simulink model "SIMULINK_1-03"  (R2024b)
settings: Solver=ode45  StartTime=0.0  StopTime=1000  RelTol=1e-7  EnableMultiTasking=on
undefined symbols (not defined in the file): gp_1, gp_2, gp_3, kc, Td, TEC, Tf, Ti
settings Model: Creator=LiberT  LastModifiedBy=Mathieu
settings SolverCC: AlgebraicLoopSolver=TrustRegion
settings DataIOCC: LimitDataPoints=on  SaveFormat=Array  SignalLoggingSaveFormat=ModelDataLogs  ReturnWorkspaceOutputs=off
settings OptimizationCC: BlockReduction=off  BooleanDataType=off  ExpressionDepthLimit=2147483647  InitFltsAndDblsToZero=on  LifeSpan=inf
settings DebuggingCC: SaveWithParameterizedLinksMsg=none  UnderspecifiedInitializationDetection=Classic  MergeDetectMultiDrivingBlocksExec=none  SignalResolutionControl=TryResolveAllWithWarning  MultiTaskDSMMsg=warning  MultiTaskCondExecSysMsg=none  FcnCallInpInsideContextMsg=warning  UnconnectedInputMsg=warning  UnconnectedOutputMsg=warning  UnconnectedLineMsg=warning  StateNameClashWarn=warning  SFUnexpectedBacktrackingDiag=warning  SFNoUnconditionalDefaultTransitionDiag=warning  SFExecutionAtInitializationDiag=none  ArithmeticOperatorsInVariantConditions=warning
settings HardwareCC: ProdBitPerPointer=32  ProdBitPerSizeT=32  ProdBitPerPtrDiffT=32  ProdLargestAtomicFloat=None  ProdIntDivRoundTo=Undefined  ProdEndianess=Unspecified  ProdWordSize=32  ProdHWDeviceType=32-bit Generic  TargetUnknown=on
settings ModelReferenceCC: EnableRefExpFcnMdlSchedulingChecks=on  PropagateSignalLabelsOutOfModel=off
settings SFSimCC: SimUseLocalCustomCode=off  CustomCodeUndefinedFunction=UseInterfaceOnly
settings RTWCC: RTWUseLocalCustomCode=off  GPUComputeCapability=3.5
settings CodeAppCC: StateflowObjectComments=on
settings GRTTargetCC: TargetFcnLib=ansi_tfl_tmw.mat  TargetLangStandard=C89/C90 (ANSI)  ModelReferenceCompliant=off  CompOptLevelCompliant=off  CombineOutputUpdateFcns=off  MatFileLogging=off  GRTInterface=on
settings ConfigComp: CovMetricSettings=dw  CovSaveCumulativeToWorkspaceVar=on  CovSaveSingleToWorkspaceVar=on  CovExternalEMLEnable=off

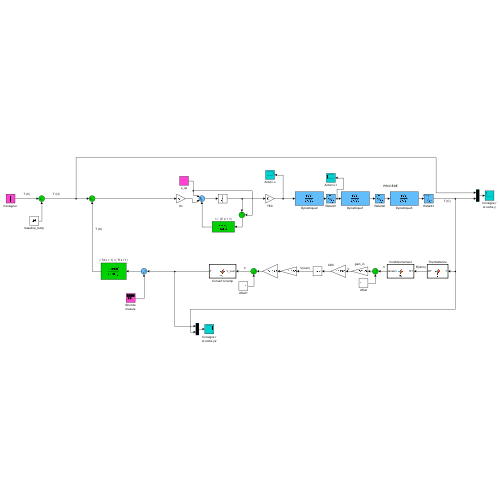
[thumbnail: Simulink's stored preview of the top-level diagram]
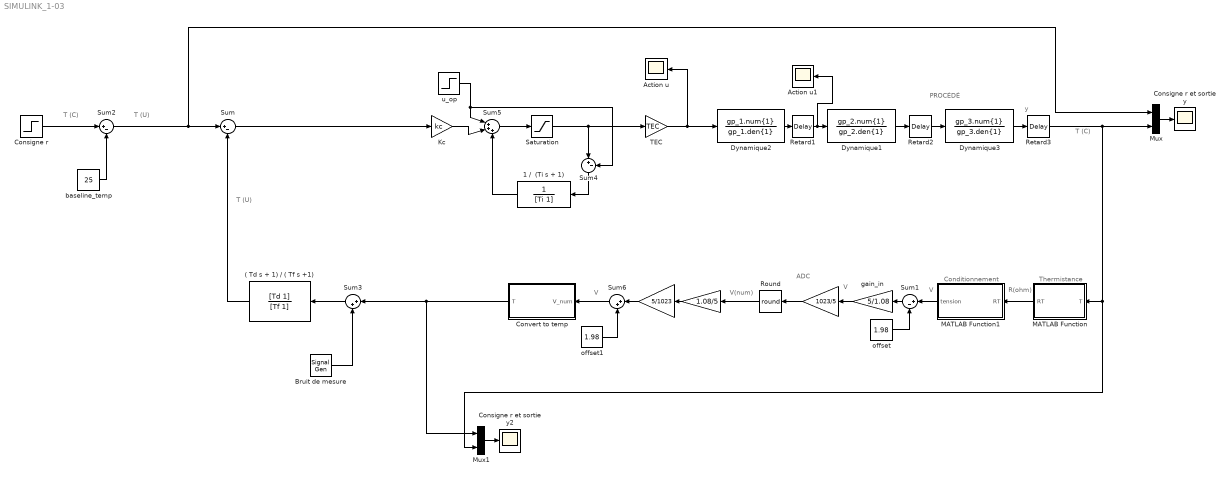
== system SIMULINK_1-03 ==
  note: T (C)
  note: PROCÉDÉ
  note: y
  note: T (U)
  note: T (U)
  note: T (C)
  note: R(ohm)
  note: V
  note: V
  note: Thermistance
  note: Conditionnement
  note: ADC
  note: V(num)
  note: V
  " " : Gain  Gain=1023/5
  "  " : Gain  Gain=1.08/5
  "   " : Gain  Gain=5/1023
  ( Td s + 1) / ( Tf s +1) : TransferFcn  Numerator=[Td 1]  Denominator=[Tf 1]
  1 /  (Ti s + 1) : TransferFcn  Numerator=1  Denominator=[Ti 1]
  Action u : Scope
  Action u1 : Scope
  Bruit de mesure : SignalGenerator  Amplitude=0  Units=rad/sec
  Consigne r : Step  Time=1000  Before=30  After=30  SampleTime=0
  Consigne r et sortie y : Scope
  Consigne r et sortie y2 : Scope
  Convert to temp : MATLAB Function  TreatAsAtomicUnit=on
  Dynamique1 : TransferFcn  Numerator=gp_2.num{1}  Denominator=gp_2.den{1}
  Dynamique2 : TransferFcn  Numerator=gp_1.num{1}  Denominator=gp_1.den{1}
  Dynamique3 : TransferFcn  Numerator=gp_3.num{1}  Denominator=gp_3.den{1}
  Kc : Gain  Gain=kc
  MATLAB Function : MATLAB Function  TreatAsAtomicUnit=on
  MATLAB Function1 : MATLAB Function  TreatAsAtomicUnit=on
  Mux : Mux  Inputs=2
  Mux1 : Mux  Inputs=2
  Retard1 : TransportDelay  DelayTime=gp_1.IODelay  BufferSize=5000
  Retard2 : TransportDelay  DelayTime=gp_2.IODelay  BufferSize=5000
  Retard3 : TransportDelay  DelayTime=gp_3.IODelay  BufferSize=5000
  Round : Rounding  Operator=round
  Saturation : Saturate  UpperLimit=1  LowerLimit=-1
  Sum{,1..2,4} (4 alike) : Sum  Inputs=|+-  InputSameDT=on  SaturateOnIntegerOverflow=on  OutDataTypeStr=Inherit: Same as first input
  Sum3 : Sum  Inputs=|++  InputSameDT=on  SaturateOnIntegerOverflow=on  OutDataTypeStr=Inherit: Same as first input
  Sum5 : Sum  Inputs=|+++  InputSameDT=on  SaturateOnIntegerOverflow=on  OutDataTypeStr=Inherit: Same as first input
  Sum6 : Sum  Inputs=|++  InputSameDT=on  SaturateOnIntegerOverflow=on  OutDataTypeStr=Inherit: Same as first input
  TEC : Gain  Gain=TEC
  baseline_temp : Constant  Value=25
  gain_in : Gain  Gain=5/1.08
  offset : Constant  Value=1.98
  offset1 : Constant  Value=1.98
  u_op : Step  Time=50  Before=0.05  After=0.05  SampleTime=0
  wires:
  Saturation/1 -> TEC/1, Sum4/1
  Retard1/1 -> Action u1/1, Dynamique1/1
  Mux/1 -> Consigne r et sortie y/1
  Sum3/1 -> ( Td s + 1) / ( Tf s +1)/1
  Bruit de mesure/1 -> Sum3/2
  Dynamique2/1 -> Retard1/1
  u_op/1 -> Sum5/1, Sum4/2
  Sum4/1 -> 1 /  (Ti s + 1)/1
  1 /  (Ti s + 1)/1 -> Sum5/3
  Sum5/1 -> Saturation/1
  Kc/1 -> Sum5/2
  Sum/1 -> Kc/1
  ( Td s + 1) / ( Tf s +1)/1 -> Sum/2
  Consigne r/1 -> Sum2/1
  baseline_temp/1 -> Sum2/2
  TEC/1 -> Dynamique2/1, Action u/1
  Dynamique1/1 -> Retard2/1
  Retard2/1 -> Dynamique3/1
  Dynamique3/1 -> Retard3/1
  Retard3/1 -> Mux1/2, MATLAB Function/1(T), Mux/2
  Sum2/1 -> Sum/1, Mux/1
  MATLAB Function/1(RT) -> MATLAB Function1/1(RT)
  MATLAB Function1/1(tension) -> Sum1/1
  offset/1 -> Sum1/2
  Sum1/1 -> gain_in/1
  "   "/1 -> Sum6/1
  offset1/1 -> Sum6/2
  gain_in/1 -> " "/1
  " "/1 -> Round/1
  Round/1 -> "  "/1
  "  "/1 -> "   "/1
  Sum6/1 -> Convert to temp/1(V_num)
  Convert to temp/1(T) -> Mux1/1, Sum3/1
  Mux1/1 -> Consigne r et sortie y2/1

== matlab function SIMULINK_1-03/MATLAB Function ==
  data: T input; RT output
function RT = r2t(T)
% Définition des coefficients
A = -14.65719769;
B = 4798.84200000;
C = -115334.00000000;
D = -3730535.00000000;
R25 = 10000; % Exemple de R25 (à adapter selon ton besoin)

% Calcul de la résistance
RT = R25 * exp(A + B./(T+273.15) + C./(T+273.15).^2 + D./(T+273.15).^3);
end

== matlab function SIMULINK_1-03/Convert to temp ==
  data: V_num input; T output
function T = v2t(V_num)
% Définition des coefficients
Rfixe = 10000;
RT = Rfixe * (5.0 /V_num - 1.0);
R25 = 10000;
lnR = log(RT / R25);   
A = 0.00335401643468053;
B = 0.000256523550896126;
C = 0.00000260597012072052;
D = 0.000000063292612648746;
T = 1.0 / (A + B * lnR + C * lnR * lnR + D * lnR * lnR * lnR) - 273.15;
end

== matlab function SIMULINK_1-03/MATLAB Function1 ==
  data: RT input; tension output
function tension = r2v(RT)
% Définition des coefficients
Rfixe = 10000;
tension = 5*(RT)/(RT+Rfixe);
end
